simulink model "Typical_second_order_system"  (R2025a)
settings: Solver=VariableStepAuto  StartTime=0.0  StopTime=5  RelTol=1e-3
InitFcn:
  | Wn = 10;
  | zeta = 0.4;
  | T = 0.001
undefined symbols (not defined in the file): dspblkCoreblockFVToolHelper, gcbh
settings Model: Creator=星必尘Sguan  LastModifiedBy=星必尘Sguan
settings SFSimCC: SimCustomHeaderCode="#include \"Damping_Loop.h\""  SimCustomInitializer=Damping_Init();  SimUserSources=Damping_Loop.c

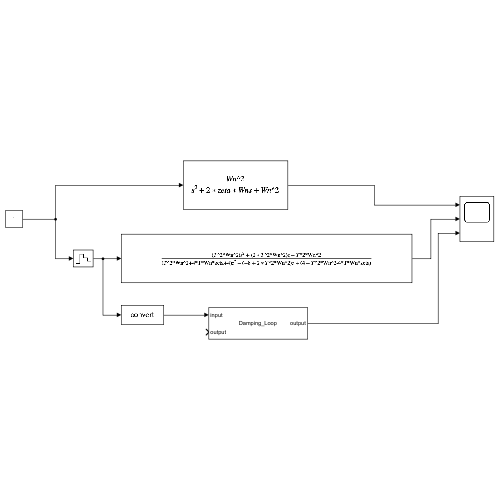
[thumbnail: Simulink's stored preview of the top-level diagram]
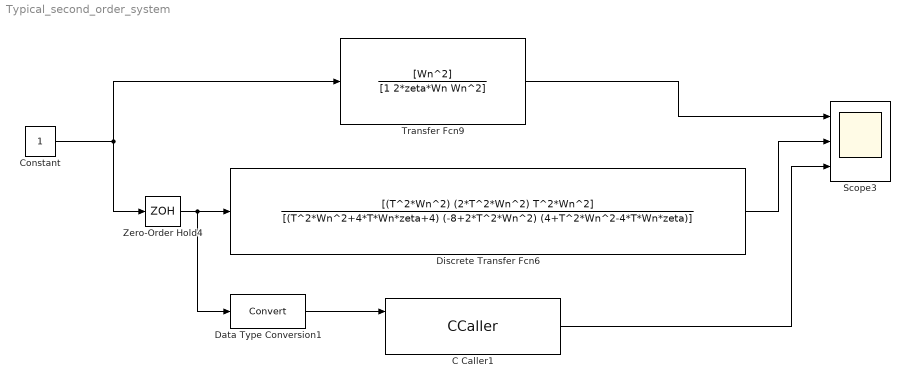
== system Typical_second_order_system ==
  C Caller1 : CCaller  FunctionName=Damping_Loop  PortSpecificationStruct="%)30     .    X ,   8    (     @         %    \"     (    !     0         %  0 \"0    $    _    07)G3F%M90  4&]R=$YA;64 4V-O<&4     26YD97@     5'EP90      4VEZ90      27-';&]B86P   X    X    !@    @    $          4    (     0    4    !         !     %    :6YP=70    .    .     8    (    !          %    \"     $    %     0         0    !0   &EN<'5T    #@   #@    &    \"     0         !0    @    !    !0    $         $     4   !);G!U=     X    X    !@    @    &          4    (     0    $    !          D    (               .    .     8    (    !          %    \"     $    &     0         0    !@   '-I;F=L90  #@   #     &    \"     0         !0    @    !     0    $         $  ! #$    .    ,     8    (    \"0(        %    \"     $    !     0         \"  $       X    X    !@    @    $          4    (     0    8    !         !     &    ;W5T<'5T   .    .     8    (    !          %    \"     $    &     0         0    !@   &]U='!U=   #@   $     &    \"     0         !0    @    !    \"P    $         $     L   !);G!U=$]U='!U=       #@   #@    &    \"     8         !0    @    !     0    $         \"0    @           #P/PX    X    !@    @    $          4    (     0    8    !         !     &    <VEN9VQE   .    ,     8    (    !          %    \"     $    \"     0         0  ( +3$   X    P    !@    @    ) @        4    (     0    $    !          (  0"
  Constant : Constant
  Data Type Conversion1 : DataTypeConversion  SaturateOnIntegerOverflow=off  RndMeth=Floor
  Discrete Transfer Fcn6 : DiscreteTransferFcn  LoadFcn=dspblkCoreblockFVToolHelper(gcbh,'load');  Numerator=[(T^2*Wn^2) (2*T^2*Wn^2) T^2*Wn^2]  Denominator=[(T^2*Wn^2+4*T*Wn*zeta+4) (-8+2*T^2*Wn^2) (4+T^2*Wn^2-4*T*Wn*zeta)]
      settings: CopyFcn=dspblkCoreblockFVToolHelper(gcbh,'copy');  DeleteFcn=dspblkCoreblockFVToolHelper(gcbh,'close');  ModelCloseFcn=dspblkCoreblockFVToolHelper(gcbh,'close');  PreSaveFcn=dspblkCoreblockFVToolHelper(gcbh,'presave');  PostSaveFcn=dspblkCoreblockFVToolHelper(gcbh,'postsave');  CloseFcn=dspblkCoreblockFVToolHelper(gcbh,'close');
  Scope3 : Scope  NumInputPorts=3
      settings: ActiveDisplayYMinimum=-0.24415285715070134  ActiveDisplayYMaximum=1.2254615103638327  DataLoggingVariableName=ScopeData3
  Transfer Fcn9 : TransferFcn  Numerator=[Wn^2]  Denominator=[1 2*zeta*Wn Wn^2]
  Zero-Order Hold4 : ZeroOrderHold  SampleTime=0.001
  wires:
  Transfer Fcn9/1 -> Scope3/1
  Discrete Transfer Fcn6/1 -> Scope3/2
  C Caller1/1 -> Scope3/3
  Data Type Conversion1/1 -> C Caller1/1
  Zero-Order Hold4/1 -> Data Type Conversion1/1, Discrete Transfer Fcn6/1
  Constant/1 -> Zero-Order Hold4/1, Transfer Fcn9/1
